simulink model "DynamicModel"  (R2016b)
settings: configuration reference "WheelSimConfiguration2016" (kept outside this file)
settings Model: Creator=At  LastModifiedBy=At
settings ConfigSetRef: SourceLocation=Base Workspace

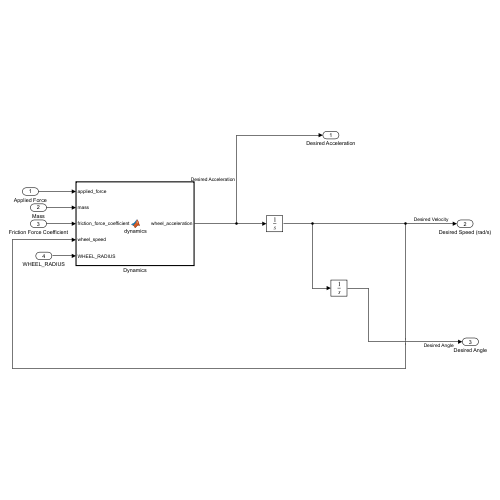
[thumbnail: Simulink's stored preview of the top-level diagram]
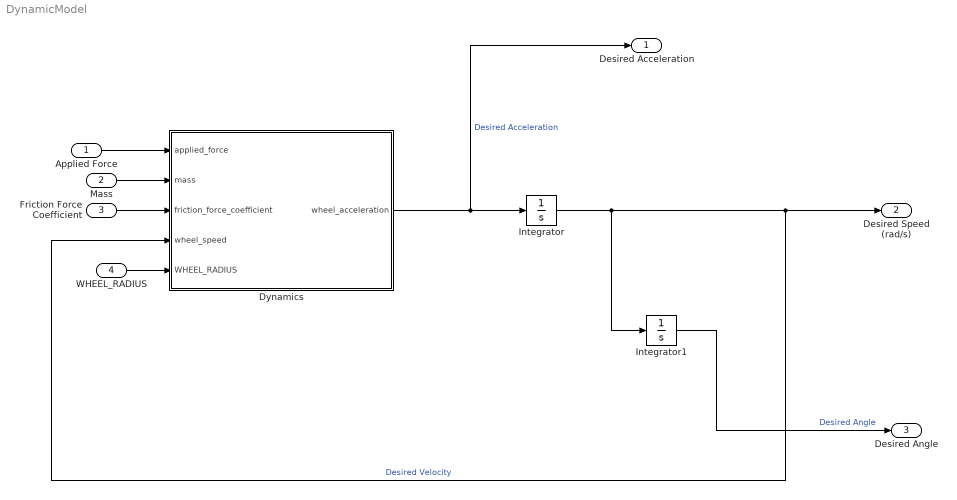
== system DynamicModel ==
  Applied Force : Inport
  Mass : Inport  Port=2
  Friction Force Coefficient : Inport  Port=3
  WHEEL_RADIUS : Inport  Port=4
  Dynamics : MATLAB Function  TreatAsAtomicUnit=on
  Integrator : Integrator
  Integrator1 : Integrator
  Desired Acceleration : Outport
  Desired Speed (rad/s) : Outport  Port=2
  Desired Angle : Outport  Port=3
  wires:
  Dynamics/1(wheel_acceleration) -> Desired Acceleration/1, Integrator/1  "Desired Acceleration"
  Integrator/1 -> Desired Speed (rad/s)/1, Dynamics/4(wheel_speed), Integrator1/1  "Desired Velocity"
  Integrator1/1 -> Desired Angle/1  "Desired Angle"
  WHEEL_RADIUS/1 -> Dynamics/5(WHEEL_RADIUS)
  Friction Force Coefficient/1 -> Dynamics/3(friction_force_coefficient)
  Mass/1 -> Dynamics/2(mass)
  Applied Force/1 -> Dynamics/1(applied_force)

== matlab function DynamicModel/Dynamics ==
  data: applied_force input; wheel_acceleration output; mass input; friction_force_coefficient input; wheel_speed input; WHEEL_RADIUS input
function wheel_acceleration  = dynamics(applied_force, mass, friction_force_coefficient, wheel_speed, WHEEL_RADIUS)

%% This function calculates the wheel acceleration based on the simple dynamic model of propelling in a straight line

g=9.81;

friction_force=friction_force_coefficient*mass*g;

wheelchair_linear_acceleration = (applied_force - (friction_force * sign(wheel_speed))) / mass;

wheel_acceleration = wheelchair_linear_acceleration / WHEEL_RADIUS;
